simulink model "model"  (R2024a)
settings: Solver=ode3  StartTime=0.0  StopTime=Tfinal  FixedStep=step_size  MaxStep=0.001  RelTol=1e-3  EnableMultiTasking=on
values from neighbouring files (symbols this model uses):
  init_cond = [0, 0, 10*pi/180, 0]    [cart_pendulum_model.m]    (also in cart_pendulum_model_angle_only_output.m = [0; 0; 10*pi/180; 0])
  step_size = .01    (= 0.01)    [cart_pendulum_model.m]    (also in cart_pendulum_model_angle_only_output.m)
  theta_variance = 5*pi/180    (= 0.0872664625997)    [cart_pendulum_model.m]    (also in cart_pendulum_model_angle_only_output.m)
  x_variance = .05    (= 0.05)    [cart_pendulum_model.m]
undefined symbols (not defined in the file or in its folder): gaussian
libraries: simulink x2
settings Model: Creator=hurstj  LastModifiedBy=Robert
settings SolverCC: AlgebraicLoopSolver=TrustRegion
settings DataIOCC: LimitDataPoints=on  SaveFormat=Array  SignalLoggingSaveFormat=ModelDataLogs  ReturnWorkspaceOutputs=off
settings OptimizationCC: ExpressionDepthLimit=2147483647  LifeSpan=inf
settings DebuggingCC: UnderspecifiedInitializationDetection=Classic  MergeDetectMultiDrivingBlocksExec=none  SolverPrmCheckMsg=warning  FcnCallInpInsideContextMsg=warning  UnconnectedInputMsg=warning  UnconnectedOutputMsg=warning  UnconnectedLineMsg=warning  StateNameClashWarn=warning  SFUnexpectedBacktrackingDiag=warning  SFNoUnconditionalDefaultTransitionDiag=warning  SFExecutionAtInitializationDiag=none  ArithmeticOperatorsInVariantConditions=warning
settings HardwareCC: ProdBitPerPointer=32  ProdBitPerSizeT=32  ProdBitPerPtrDiffT=32  ProdLargestAtomicFloat=None  ProdIntDivRoundTo=Undefined  ProdEndianess=Unspecified  ProdWordSize=32  ProdHWDeviceType=32-bit Generic
settings ModelReferenceCC: EnableRefExpFcnMdlSchedulingChecks=on  PropagateSignalLabelsOutOfModel=off
settings SFSimCC: SimUseLocalCustomCode=off  CustomCodeUndefinedFunction=UseInterfaceOnly
settings RTWCC: RTWUseLocalCustomCode=off  GPUComputeCapability=3.5  DLArmComputeVersion=19.05
settings CodeAppCC: StateflowObjectComments=on
settings GRTTargetCC: TargetLangStandard=C89/C90 (ANSI)
settings ConfigComp: CovMetricSettings=dw  CovSaveCumulativeToWorkspaceVar=on  CovSaveSingleToWorkspaceVar=on  CovExternalEMLEnable=off

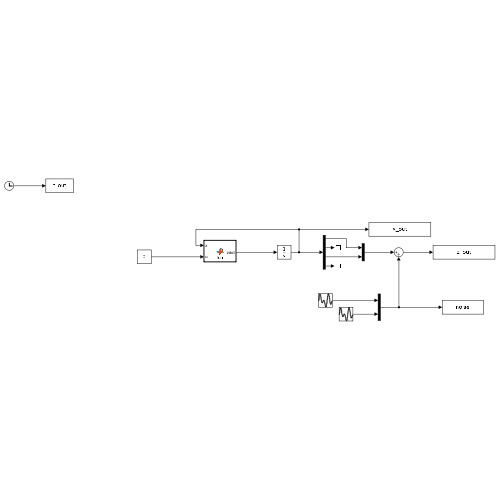
[thumbnail: Simulink's stored preview of the top-level diagram]
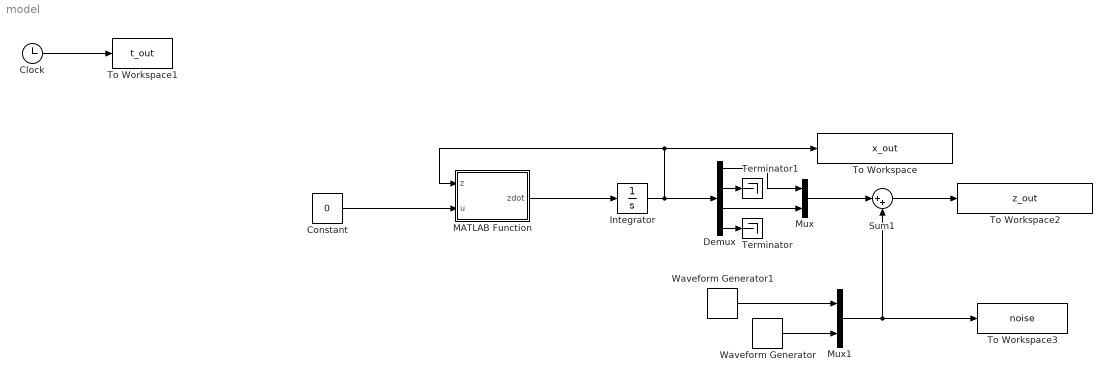
== system model ==
  Clock : Clock
  Constant : Constant  Value=0
  Demux : Demux
  Integrator : Integrator  InitialCondition=init_cond
  MATLAB Function : MATLAB Function  TreatAsAtomicUnit=on
  Mux : Mux  Inputs=2
  Mux1 : Mux  Inputs=2
  Sum1 : Sum  Inputs=|++
  Terminator : Terminator
  Terminator1 : Terminator
  To Workspace : ToWorkspace  VariableName=x_out  SaveFormat=Timeseries  SampleTime=-1
  To Workspace1 : ToWorkspace  VariableName=t_out  SampleTime=-1
  To Workspace2 : ToWorkspace  VariableName=z_out  SaveFormat=Timeseries  SampleTime=-1
  To Workspace3 : ToWorkspace  VariableName=noise  SaveFormat=Timeseries  SampleTime=-1
  Waveform Generator : simulink/Sources/Waveform Generator  OutMin=[]  OutMax=[]  OutDataTypeStr=double  SelectedSignal=1  Signals=gaussian(0,theta_variance,0)  BlockNames=MultiportSwitch_59a1d59f57604ef  SampleTime=step_size
  Waveform Generator1 : simulink/Sources/Waveform Generator  OutMin=[]  OutMax=[]  OutDataTypeStr=double  SelectedSignal=1  Signals=gaussian(0,x_variance,0)  BlockNames=MultiportSwitch_f67fa682d7ac4fa  SampleTime=step_size
  wires:
  Clock/1 -> To Workspace1/1
  Integrator/1 -> Demux/1, MATLAB Function/1(z), To Workspace/1
  Constant/1 -> MATLAB Function/2(u)
  MATLAB Function/1(zdot) -> Integrator/1
  Demux/1 -> Mux/1
  Demux/3 -> Mux/2
  Mux/1 -> Sum1/1
  Sum1/1 -> To Workspace2/1
  Demux/2 -> Terminator1/1
  Demux/4 -> Terminator/1
  Mux1/1 -> Sum1/2, To Workspace3/1
  Waveform Generator1/1 -> Mux1/1
  Waveform Generator/1 -> Mux1/2

== matlab function model/MATLAB Function ==
  data: z input size=4; u input; zdot output size=4
function zdot = fcn(z,u)
zdot=zeros(4,1);
mb=2.3;
mp=1.4;
l=.88;
g=9.8;
Bp=.0178;
Bb=.734;
M=[mp+mb,           -mp*l*cos(z(3));
   -mp*l*cos(z(3)), mp*l^2];
b=[u - mp*l*sin(z(3))*z(4)^2-Bb*z(2);
    mp*g*l*sin(z(3))-Bp*z(4)];
temp=M^-1*b;

zdot(1)=z(2);
zdot(2)=temp(1);
zdot(3)=z(4);
zdot(4)=temp(2);
end
